simulink library "MagnetoLibrary"  (R2019a)
settings: Solver=VariableStepAuto  StartTime=0.0  StopTime=10.0  RelTol=1e-3
undefined symbols (not defined in the file or in its folder): quantity, Ts
libraries: arduinolib x8, $bdroot x4
settings Model: Creator=Jakub  LastModifiedBy=Jakub

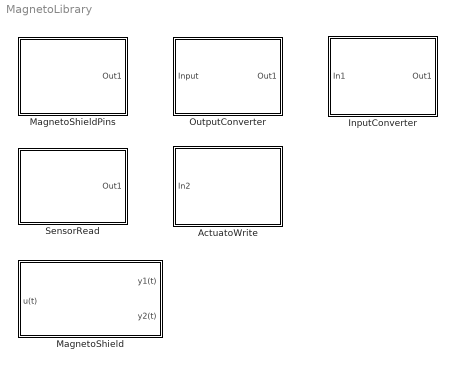
== system MagnetoLibrary ==
  ActuatoWrite : Subsystem  mask{Board=UNO/MEGA, Units=Volts}
      mask prompts: Board "Type of the Arduino board"; Units "Input unite"
      mask help:
      | ActuatorWrite block allows to set desired voltage value on the electromagnet. The desired value can be expresed as voltage, percentage of maximal possible voltage or as a value of the magnetic field in Gausses as well.
      | This block converts input control signal into suficient form (16-bit number) and writes the information on the MCP4725-DAC converter.
      | Maximal voltage range: 0-12 V
      mask init:
      | mask_popup = get_param(gcb,'Board'); % which popup is choosen
      | % path to the I2C Write block
      | system = gcb;
      | way = strcat(system,'/I2C Write UNO');
      | % set Module based on Arduino type
      | if strcmp(mask_popup(1),'U')
      |     set_param(way,'I2CModule','0'); % Uno/Mega - module 0
      | elseif strcmp(mask_popup(1),'D')
      |     set_param(way,'I2CModule','1'); % Due - module 1
      | end
      settings: CopyFcn=set_param(gcb, 'LinkStatus', 'inactive')
      mask TypeOptions Board: UNO/MEGA | DUE
      mask TypeOptions Units: Volts | Percents | DAC levels
      mask DialogControl DescGroupVar Prompt: ActuatorWrite block
      mask Display: image('assets\MagnetoFig\ActuatorWrite.bmp');
  InputConverter : Subsystem  mask{Units=Percents}
      mask prompts: Units "Choos input unit"
      mask help:
      | This block provide conversion between choosen input units and convert it into double number in range 0 to 4095. This converted size is suitable for "ActuatorWrite" block.
      | (input = double/output = double)
      mask init:
      | if Units==1
      | path = 'assets\MagnetoFig\InputCon\VtoDAC.bmp';
      | elseif Units==2
      | path = 'assets\MagnetoFig\InputCon\PERtoDAC.bmp';
      | else
      | path = 'assets\MagnetoFig\InputCon\DACtoDAC.bmp';    
      | end
      mask TypeOptions Units: Voltage | Percents | DAC levels
      mask DialogControl DescGroupVar Prompt: InputConverter block
      mask Display: image(path);
  MagnetoShield : Subsystem  mask{Board=UNO/MEGA, PositionType=Distance [mm], chackbox=on, Ts=0.001}
      mask prompts: Board "Type of the Arduino board"; PositionType "Position measured in:"; chackbox "Execute calibration at the biginning of the simulation"; Ts "Sampling period [s]"
      settings: CopyFcn=set_param(gcb, 'LinkStatus', 'inactive')
      mask TypeOptions Board: UNO/MEGA | DUE
      mask TypeOptions PositionType: Distance [mm] | Percents [%]
      mask DialogControl ParameterGroupVar Prompt: Arduino board
  MagnetoShieldPins : Subsystem  mask{PIN=Hall sensor pin (A3), sampling=0.001}
      mask prompts: PIN "Choose pin"; sampling "Sampling period [s]"
      mask help:
      | User can choose a pin on which the data should be processed.
      | >Hall sensor pin - data about the possition of the levitating magnet.
      | >Voltage pin - voltage on the electromagnet
      | >Current pin - current crossing the electromagnet
      | >Reference pin - data from potentiometer, used as adjustable analog reference
      | (output = double)
      mask init:
      | letter = PIN;
      | if letter==1
      | path='assets\MagnetoFig\Pins\hpin.bmp';
      | elseif letter==2
      | path='assets\MagnetoFig\Pins\vpin.bmp';
      | elseif letter==3
      | path='assets\MagnetoFig\Pins\cpin.bmp';
      | else
      | path='assets\MagnetoFig\Pins\ppin.bmp';    
      | end
      settings: CopyFcn=set_param(gcb, 'LinkStatus', 'inactive')
      mask TypeOptions PIN: Hall sensor pin (A3) | Voltage pin (A1) | Current pin (A2) | Reference pin (A0)
      mask Callback PIN:
      | mask_popup = get_param(gcb,'PIN'); % which popup is choosen
      | % path to the I2C Write block
      | system = gcb;
      | way = strcat(system,'/Analog Input');
      | % set Module based on Arduino type
      | if strcmp(mask_popup(1),'H')
      |     set_param(way,'pinNumber','3'); % Uno/Mega - module 0
      | elseif strcmp(mask_popup(1),'V')
      |     set_param(way,'pinNumber','1'); % Due - module 1
      | elseif strcmp(mask_popup(1),'C')
      |     set_param(way,'pinNumber','2'); % Due - module 1
      | elseif strcmp(mask_popup(1),'R')
      |     set_param(way,'pinNumber','0'); % Due - module 11
      | end
      mask DialogControl DescGroupVar Prompt: MagnetoShieldPins block
      mask Display: image(path);
  OutputConverter : Subsystem  mask{BoardType=UNO/MEGA, Units=Position, Pos=Distance, Dconst1=3.233100, Dconst2=0.220571, ADCmin_UNO=27, ADCmax_UNO=776, ADCmin_DUE=100, ADCmax_DUE=2315, ChackBox=off, VoltGain=4, CurrGain=33.333333, Parameter13=on}
      mask prompts: BoardType "Type of the Arduino board"; Units "Measured quantity"; Pos "Position unites"; Dconst1 "Position constant 1"; Dconst2 "Position constant 2"; ADCmin_UNO "Minimal ADC value uno"; ADCmax_UNO "Maximal  ADC value uno"; ADCmin_DUE "Minimal ADC value"; ADCmax_DUE "Maximal  ADC value"; ChackBox "Advanced options"; VoltGain "Voltage gain"; CurrGain "Current gain"; Parameter13 "Len pre funkcionalitu"
      mask help:
      | This block converts output signal from the system into choosen physical unit.
      | Entering signal is in the form of 8-bit number for Arduino UNO/MEGA or 12-bit number for Arduino DUE. Value on the output is defined by the choosen unit and possibly by the adjustnemts of these quantities.
      | Prefered input values from "MagnetoShieldPins" block.
      | (input = double/output = double)
      mask init:
      | if Units == 1 %position
      |         if Pos == 1 %mm
      |             path = 'assets\MagnetoFig\OutputCon\ADCtoMM.bmp'
      |         elseif Pos == 2 % percents
      |             path = 'assets\MagnetoFig\OutputCon\ADCtoPer.bmp'
      |         elseif Pos == 3 %gauss
      |            path = 'assets\MagnetoFig\OutputCon\ADCtoGauss.bmp' 
      |         else % adc levels
      |             path = 'assets\MagnetoFig\OutputCon\ADCtoADC.bmp'
      |         end
      |     elseif Units == 2 %voltage
      |         path = 'assets\MagnetoFig\OutputCon\ADCtoVolt.bmp'
      |     elseif Units == 3 %current
      |         path = 'assets\MagnetoFig\OutputCon\ADCtoAmp.bmp'
      |     else %analog reference
      |         path = 'assets\MagnetoFig\OutputCon\ADCtoRef.bmp'
      |     end
      mask TypeOptions BoardType: UNO/MEGA | DUE
      mask Callback BoardType:
      | mask_popup = get_param(gcb,'Units'); %Vyber meranej veliciny - Napatie/Prud/Poloha/Referencia
      | 
      | if strcmp(mask_popup(1),'P') %Ak meriam polohu
      |     set_param(gcb,'MaskVisibilities',{'on','on','on','off','off','off','off','off','off','off','off','off','off'});
      |     MeassurePos = get_param(gcb,'Pos'); %V com meriam polohu - Gauss/Vyska/Percenta/ADC
      |     if strcmp(MeassurePos(1),'D')
      |         set_param(gcb,'MaskVisibilities',{'on','on','on','on','on','off','off','off','off','off','off','off','off'});
      |     elseif strcmp(MeassurePos(1),'P')
      |         TypeOfBoard = get_param(gcb,'BoardType'); %Ak meriam v %, aku mam dosku?
      |         if strcmp(TypeOfBoard(1),'U')
      |             set_param(gcb,'MaskVisibilities',{'on','on','on','off','off','on','on','off','off','off','off','off','off'});
      |         else
      |             set_param(gcb,'MaskVisibilities',{'on','on','on','off','off','off','off','on','on','off','off','off','off'});
      |         end
      |     elseif strcmp(MeassurePos(1),'G')
      |         set_param(gcb,'MaskVisibilities',{'on','on','on','off','off','off','off','off','off','off','off','off','off'});
      |     else
      |         set_param(gcb,'MaskVisibilities',{'on','on','on','off','off','off','off','off','off','off','off','off','off'});
      |     end
      | elseif strcmp(mask_popup(1),'V') %Ak meriam napatie
      |     set_param(gcb,'MaskVisibilities',{'on','on','off','off','off','off','off','off','off','on','off','off','off'});
      |     mask_popupV = get_param(gcb,'ChackBox');
      |     if strcmp(mask_popupV(1),'o') & strcmp(mask_popupV(2),'n')%mask_popup == 'on'
      |         set_param(gcb,'MaskVisibilities',{'on','on','off','off','off','off','off','off','off','on','on','on','off'});
      |     else
      |         set_param(gcb,'MaskVisibilities',{'on','on','off','off','off','off','off','off','off','on','off','off','off'});
      |     end
      | elseif strcmp(mask_popup(1),'C') %Ak meriam prud
      |     set_param(gcb,'MaskVisibilities',{'on','on','off','off','off','off','off','off','off','on','off','off','off'});
      |     mask_popupC = get_param(gcb,'ChackBox');
      |     if strcmp(mask_popupC(1),'o') & strcmp(mask_popupC(2),'n')%mask_popup == 'on'
      |         set_param(gcb,'MaskVisibilities',{'on','on','off','off','off','off','off','off','off','on','on','on','off'});
      |     else
      |         set_param(gcb,'MaskVisibilities',{'on','on','off','off','off','off','off','off','off','on','off','off','off'});
      |     end
      | else %Ak meriam referenciu
      |     set_param(gcb,'MaskVisibilities',{'on','on','off','off','off','off','off','off','off','off','off','off','off'});
      | end
      mask TypeOptions Units: Position | Voltage [V] | Current [mA] | Analog reference [%]
      mask Callback Units:
      | mask_popup = get_param(gcb,'Units'); %Vyber meranej veliciny - Napatie/Prud/Poloha/Referencia
      | 
      | if strcmp(mask_popup(1),'P') %Ak meriam polohu
      |     set_param(gcb,'MaskVisibilities',{'on','on','on','off','off','off','off','off','off','off','off','off','off'});
      |     MeassurePos = get_param(gcb,'Pos'); %V com meriam polohu - Gauss/Vyska/Percenta/ADC
      |     if strcmp(MeassurePos(1),'D')
      |         set_param(gcb,'MaskVisibilities',{'on','on','on','on','on','off','off','off','off','off','off','off','off'});
      |     elseif strcmp(MeassurePos(1),'P')
      |         TypeOfBoard = get_param(gcb,'BoardType'); %Ak meriam v %, aku mam dosku?
      |         if strcmp(TypeOfBoard(1),'U')
      |             set_param(gcb,'MaskVisibilities',{'on','on','on','off','off','on','on','off','off','off','off','off','off'});
      |         else
      |             set_param(gcb,'MaskVisibilities',{'on','on','on','off','off','off','off','on','on','off','off','off','off'});
      |         end
      |     elseif strcmp(MeassurePos(1),'G')
      |         set_param(gcb,'MaskVisibilities',{'on','on','on','off','off','off','off','off','off','off','off','off','off'});
      |     else
      |         set_param(gcb,'MaskVisibilities',{'on','on','on','off','off','off','off','off','off','off','off','off','off'});
      |     end
      | elseif strcmp(mask_popup(1),'V') %Ak meriam napatie
      |     set_param(gcb,'MaskVisibilities',{'on','on','off','off','off','off','off','off','off','on','off','off','off'});
      |     mask_popupV = get_param(gcb,'ChackBox');
      |     if strcmp(mask_popupV(1),'o') & strcmp(mask_popupV(2),'n')%mask_popup == 'on'
      |         set_param(gcb,'MaskVisibilities',{'on','on','off','off','off','off','off','off','off','on','on','on','off'});
      |     else
      |         set_param(gcb,'MaskVisibilities',{'on','on','off','off','off','off','off','off','off','on','off','off','off'});
      |     end
      | elseif strcmp(mask_popup(1),'C') %Ak meriam prud
      |     set_param(gcb,'MaskVisibilities',{'on','on','off','off','off','off','off','off','off','on','off','off','off'});
      |     mask_popupC = get_param(gcb,'ChackBox');
      |     if strcmp(mask_popupC(1),'o') & strcmp(mask_popupC(2),'n')%mask_popup == 'on'
      |         set_param(gcb,'MaskVisibilities',{'on','on','off','off','off','off','off','off','off','on','on','on','off'});
      |     else
      |         set_param(gcb,'MaskVisibilities',{'on','on','off','off','off','off','off','off','off','on','off','off','off'});
      |     end
      | else %Ak meriam referenciu
      |     set_param(gcb,'MaskVisibilities',{'on','on','off','off','off','off','off','off','off','off','off','off','off'});
      | end
      mask TypeOptions Pos: Distance | Percents | Gauss | ADC levels
      mask Callback Pos:
      | MeassurePos = get_param(gcb,'Pos'); %V com meriam polohu - Gauss/Vyska/Percenta/ADC
      |     if strcmp(MeassurePos(1),'D')
      |         set_param(gcb,'MaskVisibilities',{'on','on','on','on','on','off','off','off','off','off','off','off','off'});
      |     elseif strcmp(MeassurePos(1),'P')
      |         TypeOfBoard = get_param(gcb,'BoardType'); %Ak meriam v %, aku mam dosku?
      |         if strcmp(TypeOfBoard(1),'U')
      |             set_param(gcb,'MaskVisibilities',{'on','on','on','off','off','on','on','off','off','off','off','off','off'});
      |         else
      |             set_param(gcb,'MaskVisibilities',{'on','on','on','off','off','off','off','on','on','off','off','off','off'});
      |         end
      |     elseif strcmp(MeassurePos(1),'G')
      |         set_param(gcb,'MaskVisibilities',{'on','on','on','off','off','off','off','off','off','off','off','off','off'});
      |     else
      |         set_param(gcb,'MaskVisibilities',{'on','on','on','off','off','off','off','off','off','off','off','off','off'});
      |     end
      mask Callback ChackBox:
      | mask_popup = get_param(gcb,'ChackBox');
      | 
      | if strcmp(mask_popup(1),'o') & strcmp(mask_popup(2),'n')%mask_popup == 'on'
      |     set_param(gcb,'MaskVisibilities',{'on','on','off','off','off','off','off','off','off','on','on','on','off'});
      | else
      |     set_param(gcb,'MaskVisibilities',{'on','on','off','off','off','off','off','off','off','on','off','off','off'});
      | end
      mask Callback Parameter13:
      | mask_popup = get_param(gcb,'Units'); %Vyber meranej veliciny - Napatie/Prud/Poloha/Referencia
      | 
      | if strcmp(mask_popup(1),'P') %Ak meriam polohu
      |     set_param(gcb,'MaskVisibilities',{'on','on','on','off','off','off','off','off','off','off','off','off','off'});
      |     MeassurePos = get_param(gcb,'Pos'); %V com meriam polohu - Gauss/Vyska/Percenta/ADC
      |     if strcmp(MeassurePos(1),'D')
      |         set_param(gcb,'MaskVisibilities',{'on','on','on','on','on','off','off','off','off','off','off','off','off'});
      |     elseif strcmp(MeassurePos(1),'P')
      |         TypeOfBoard = get_param(gcb,'BoardType'); %Ak meriam v %, aku mam dosku?
      |         if strcmp(TypeOfBoard(1),'U')
      |             set_param(gcb,'MaskVisibilities',{'on','on','on','off','off','on','on','off','off','off','off','off','off'});
      |         else
      |             set_param(gcb,'MaskVisibilities',{'on','on','on','off','off','off','off','on','on','off','off','off','off'});
      |         end
      |     elseif strcmp(MeassurePos(1),'G')
      |         set_param(gcb,'MaskVisibilities',{'on','on','on','off','off','off','off','off','off','off','off','off','off'});
      |     else
      |         set_param(gcb,'MaskVisibilities',{'on','on','on','off','off','off','off','off','off','off','off','off','off'});
      |     end
      | elseif strcmp(mask_popup(1),'V') %Ak meriam napatie
      |     set_param(gcb,'MaskVisibilities',{'on','on','off','off','off','off','off','off','off','on','off','off','off'});
      |     mask_popupV = get_param(gcb,'ChackBox');
      |     if strcmp(mask_popupV(1),'o') & strcmp(mask_popupV(2),'n')%mask_popup == 'on'
      |         set_param(gcb,'MaskVisibilities',{'on','on','off','off','off','off','off','off','off','on','on','on','off'});
      |     else
      |         set_param(gcb,'MaskVisibilities',{'on','on','off','off','off','off','off','off','off','on','off','off','off'});
      |     end
      | elseif strcmp(mask_popup(1),'C') %Ak meriam prud
      |     set_param(gcb,'MaskVisibilities',{'on','on','off','off','off','off','off','off','off','on','off','off','off'});
      |     mask_popupC = get_param(gcb,'ChackBox');
      |     if strcmp(mask_popupC(1),'o') & strcmp(mask_popupC(2),'n')%mask_popup == 'on'
      |         set_param(gcb,'MaskVisibilities',{'on','on','off','off','off','off','off','off','off','on','on','on','off'});
      |     else
      |         set_param(gcb,'MaskVisibilities',{'on','on','off','off','off','off','off','off','off','on','off','off','off'});
      |     end
      | else %Ak meriam referenciu
      |     set_param(gcb,'MaskVisibilities',{'on','on','off','off','off','off','off','off','off','off','off','off','off'});
      | end
      mask DialogControl DescGroupVar Prompt: OutputConverter block
      mask DialogControl ParameterGroupVar Prompt: Arduino board
      mask DialogControl Container3 Prompt: Parameters
      mask Display: image(path,'center');
  SensorRead : Subsystem  mask{board=UNO/MEGA, sensor=Distance [mm], sampling=0.001}
      mask prompts: board "Type of the Arduino board"; sensor "Sensor type"; sampling "Sampling period [s]"
      settings: CopyFcn=set_param(gcb, 'LinkStatus', 'inactive')
      mask TypeOptions board: UNO/MEGA | DUE
      mask TypeOptions sensor: Distance [mm] | Current [mA] | Voltage [V] | Analog reference [%]
      mask Callback sensor:
      | mask_popup = get_param(gcb,'sensor'); % which popup is choosen
      | % path to the I2C Write block
      | system = gcb;
      | way = strcat(system,'/Analog Input');
      | % set Module based on Arduino type
      | if strcmp(mask_popup(1),'D')
      |     set_param(way,'pinNumber','3');
      | elseif strcmp(mask_popup(1),'V')
      |     set_param(way,'pinNumber','1'); % Due - module 1
      | elseif strcmp(mask_popup(1),'C')
      |     set_param(way,'pinNumber','2'); % Due - module 1
      | elseif strcmp(mask_popup(1),'A')
      |     set_param(way,'pinNumber','0'); % Due - module 11
      | end
      mask DialogControl ParameterGroupVar Prompt: Arduino board

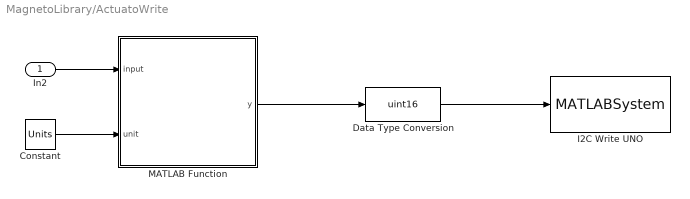
== system MagnetoLibrary/ActuatoWrite ==
  In2 : Inport
  Constant : Constant  Value=Units
  Data Type Conversion : DataTypeConversion  OutDataTypeStr=uint16
  I2C Write UNO : MATLABSystem  AncestorBlock=arduinolib/I2C Write  InitFcn=|  System=codertarget.arduinobase.internal.arduinoI2CWrite  I2CModule=0  Mode=Master  SlaveAddress=96  SlaveByteOrder=BigEndian  Direction=Transmitter  RegisterAddressMode=off  RegisterAddress=0  SlaveDataType=uint8  DataLength=1  NoAck=off  RepeatedStart=off  OutputStatus=off  blockPlatform=ARDUINO
      | codertarget.arduinobase.blocks.registerI2CBlock(gcbh);
      | codertarget.arduinobase.blocks.arduinoBlockInitFcnCallback(gcbh);
      mask Type: I2C Write
      mask Display:
      | color('white');
      | plot([100,100,100,100],[100,100,100,100]);
      | plot([0,0,0,0],[0,0,0,0]);
      | color('blue');
      | text(99, 92, 'ARDUINO', 'horizontalAlignment', 'right');
      | color('black');
      | text(50,60,'\fontsize{12}\bfI2C','texmode','on','horizontalAlignment','center','verticalAlignment','middle');
      | text(50,40,'\fontsize{10}\bfMaster Write','texmode','on','horizontalAlignment','center','verticalAlignment','middle');
      | text(50,15,'Slave: 0x60' ,'horizontalAlignment', 'center');
      | port_label('input',1,'Data');
  MATLAB Function : MATLAB Function  TreatAsAtomicUnit=on
  wires:
  In2/1 -> MATLAB Function/1(input)
  Constant/1 -> MATLAB Function/2(unit)
  Data Type Conversion/1 -> I2C Write UNO/1
  MATLAB Function/1(y) -> Data Type Conversion/1

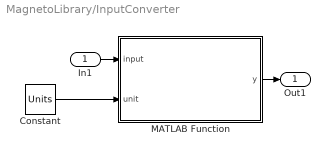
== system MagnetoLibrary/InputConverter ==
  In1 : Inport
  Constant : Constant  Value=Units
  MATLAB Function : MATLAB Function  TreatAsAtomicUnit=on
  Out1 : Outport
  wires:
  MATLAB Function/1(y) -> Out1/1
  Constant/1 -> MATLAB Function/2(unit)
  In1/1 -> MATLAB Function/1(input)

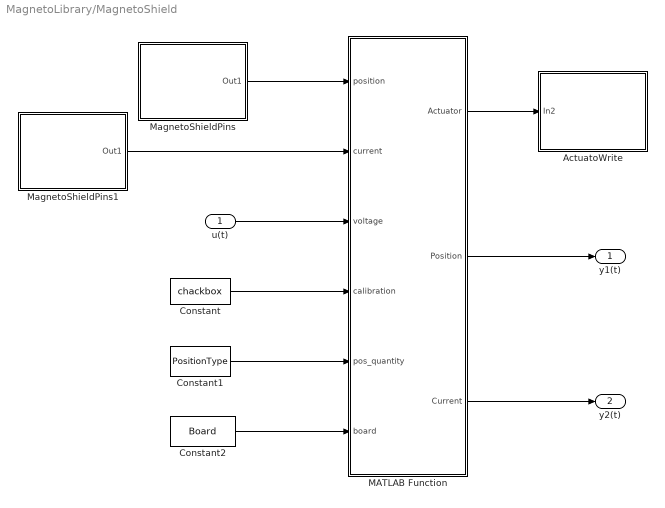
== system MagnetoLibrary/MagnetoShield ==
  u(t) : Inport
  ActuatoWrite : Subsystem  AncestorBlock=MagnetoLibrary/ActuatoWrite  mask{Board=DUE, Units=Volts}
      mask prompts: Board "Type of the Arduino board"; Units "Input unite"
      mask help:
      | ActuatorWrite block allows to set desired voltage value on the electromagnet. The desired value can be expresed as voltage, percentage of maximal possible voltage or as a value of the magnetic field in Gausses as well.
      | This block converts input control signal into suficient form (16-bit number) and writes the information on the MCP4725-DAC converter.
      | Maximal voltage range: 0-12 V
      mask init: same as MagnetoLibrary/ActuatoWrite
      settings: CopyFcn=set_param(gcb, 'LinkStatus', 'inactive')
      mask TypeOptions Board: UNO/MEGA | DUE
      mask TypeOptions Units: Volts | Percents | DAC levels
      mask DialogControl DescGroupVar Prompt: ActuatorWrite block
      mask Display: image('assets\MagnetoFig\ActuatorWrite.bmp');
  Constant : Constant  Value=chackbox  SampleTime=Ts
  Constant1 : Constant  Value=PositionType  SampleTime=Ts
  Constant2 : Constant  Value=Board  SampleTime=Ts
  MATLAB Function : MATLAB Function  TreatAsAtomicUnit=on
  MagnetoShieldPins : Subsystem  AncestorBlock=MagnetoLibrary/MagnetoShieldPins  mask{PIN=Hall sensor pin (A3), sampling=Ts}
      mask prompts: PIN "Choose pin"; sampling "Sampling period [s]"
      mask help:
      | User can choose a pin on which the data should be processed.
      | >Hall sensor pin - data about the possition of the levitating magnet.
      | >Voltage pin - voltage on the electromagnet
      | >Current pin - current crossing the electromagnet
      | >Reference pin - data from potentiometer, used as adjustable analog reference
      | (output = double)
      mask init: same as MagnetoLibrary/MagnetoShieldPins
      settings: CopyFcn=set_param(gcb, 'LinkStatus', 'inactive')
      mask TypeOptions PIN: Hall sensor pin (A3) | Voltage pin (A1) | Current pin (A2) | Reference pin (A0)
      mask Callback PIN:
      | mask_popup = get_param(gcb,'PIN'); % which popup is choosen
      | % path to the I2C Write block
      | system = gcb;
      | way = strcat(system,'/Analog Input');
      | % set Module based on Arduino type
      | if strcmp(mask_popup(1),'H')
      |     set_param(way,'pinNumber','3'); % Uno/Mega - module 0
      | elseif strcmp(mask_popup(1),'V')
      |     set_param(way,'pinNumber','1'); % Due - module 1
      | elseif strcmp(mask_popup(1),'C')
      |     set_param(way,'pinNumber','2'); % Due - module 1
      | elseif strcmp(mask_popup(1),'R')
      |     set_param(way,'pinNumber','0'); % Due - module 11
      | end
      mask DialogControl DescGroupVar Prompt: MagnetoShieldPins block
      mask Display: image(path);
  MagnetoShieldPins1 : Subsystem  AncestorBlock=MagnetoLibrary/MagnetoShieldPins  mask{PIN=Current pin (A2), sampling=Ts}
      mask prompts: PIN "Choose pin"; sampling "Sampling period [s]"
      mask help:
      | User can choose a pin on which the data should be processed.
      | >Hall sensor pin - data about the possition of the levitating magnet.
      | >Voltage pin - voltage on the electromagnet
      | >Current pin - current crossing the electromagnet
      | >Reference pin - data from potentiometer, used as adjustable analog reference
      | (output = double)
      mask init: same as MagnetoLibrary/MagnetoShieldPins
      settings: CopyFcn=set_param(gcb, 'LinkStatus', 'inactive')
      mask TypeOptions PIN: Hall sensor pin (A3) | Voltage pin (A1) | Current pin (A2) | Reference pin (A0)
      mask Callback PIN:
      | mask_popup = get_param(gcb,'PIN'); % which popup is choosen
      | % path to the I2C Write block
      | system = gcb;
      | way = strcat(system,'/Analog Input');
      | % set Module based on Arduino type
      | if strcmp(mask_popup(1),'H')
      |     set_param(way,'pinNumber','3'); % Uno/Mega - module 0
      | elseif strcmp(mask_popup(1),'V')
      |     set_param(way,'pinNumber','1'); % Due - module 1
      | elseif strcmp(mask_popup(1),'C')
      |     set_param(way,'pinNumber','2'); % Due - module 1
      | elseif strcmp(mask_popup(1),'R')
      |     set_param(way,'pinNumber','0'); % Due - module 11
      | end
      mask DialogControl DescGroupVar Prompt: MagnetoShieldPins block
      mask Display: image(path);
  y1(t) : Outport
  y2(t) : Outport  Port=2
  wires:
  MATLAB Function/3(Current) -> y2(t)/1
  Constant2/1 -> MATLAB Function/6(board)
  Constant1/1 -> MATLAB Function/5(pos_quantity)
  Constant/1 -> MATLAB Function/4(calibration)
  MagnetoShieldPins1/1(Out1) -> MATLAB Function/2(current)
  u(t)/1 -> MATLAB Function/3(voltage)
  MATLAB Function/2(Position) -> y1(t)/1
  MagnetoShieldPins/1(Out1) -> MATLAB Function/1(position)
  MATLAB Function/1(Actuator) -> ActuatoWrite/1(In2)

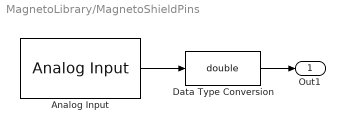
== system MagnetoLibrary/MagnetoShieldPins ==
  Analog Input : arduinolib/Analog Input  pinNumber=3  ReadResultsOnly=off  ConversionTriggerSource=Software  ExternalTriggerType=uint32(0)  OutputDataType=uint16  EnableConversionCompleteNotify=off  EnableOuputStatus=off  SampleTime=sampling  blockPlatform=arduino
  Data Type Conversion : DataTypeConversion  OutDataTypeStr=double
  Out1 : Outport
  wires:
  Analog Input/1 -> Data Type Conversion/1
  Data Type Conversion/1 -> Out1/1

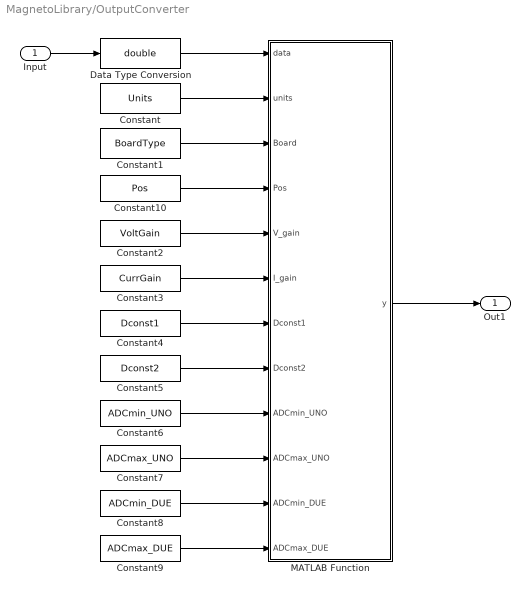
== system MagnetoLibrary/OutputConverter ==
  Input : Inport
  Constant : Constant  Value=Units
  Constant1 : Constant  Value=BoardType
  Constant10 : Constant  Value=Pos
  Constant2 : Constant  Value=VoltGain
  Constant3 : Constant  Value=CurrGain
  Constant4 : Constant  Value=Dconst1
  Constant5 : Constant  Value=Dconst2
  Constant6 : Constant  Value=ADCmin_UNO
  Constant7 : Constant  Value=ADCmax_UNO
  Constant8 : Constant  Value=ADCmin_DUE
  Constant9 : Constant  Value=ADCmax_DUE
  Data Type Conversion : DataTypeConversion  OutDataTypeStr=double
  MATLAB Function : MATLAB Function  TreatAsAtomicUnit=on
  Out1 : Outport
  wires:
  Constant4/1 -> MATLAB Function/7(Dconst1)
  Constant5/1 -> MATLAB Function/8(Dconst2)
  Constant6/1 -> MATLAB Function/9(ADCmin_UNO)
  Constant7/1 -> MATLAB Function/10(ADCmax_UNO)
  Constant8/1 -> MATLAB Function/11(ADCmin_DUE)
  Constant9/1 -> MATLAB Function/12(ADCmax_DUE)
  Data Type Conversion/1 -> MATLAB Function/1(data)
  Constant3/1 -> MATLAB Function/6(I_gain)
  Constant2/1 -> MATLAB Function/5(V_gain)
  Constant1/1 -> MATLAB Function/3(Board)
  Constant/1 -> MATLAB Function/2(units)
  MATLAB Function/1(y) -> Out1/1
  Input/1 -> Data Type Conversion/1
  Constant10/1 -> MATLAB Function/4(Pos)

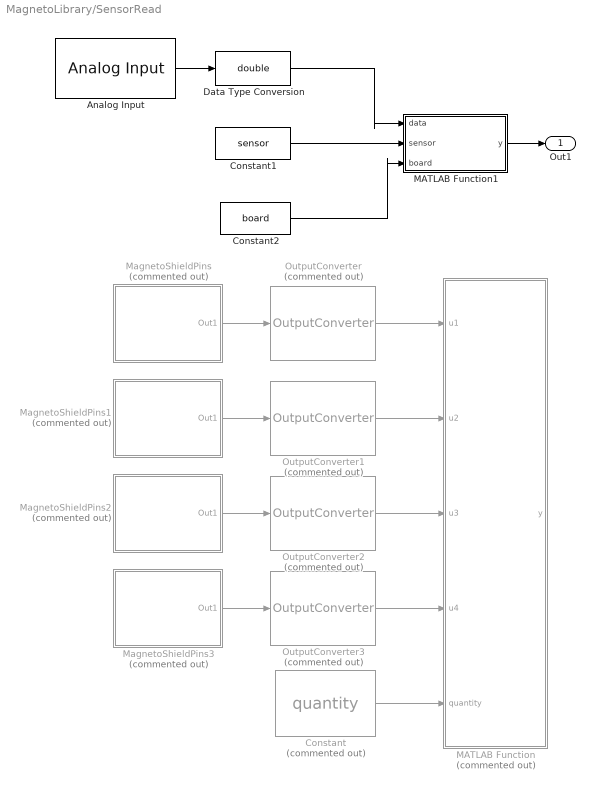
== system MagnetoLibrary/SensorRead ==
  Analog Input : arduinolib/Analog Input  pinNumber=3  ReadResultsOnly=off  ConversionTriggerSource=Software  ExternalTriggerType=uint32(0)  OutputDataType=uint16  EnableConversionCompleteNotify=off  EnableOuputStatus=off  SampleTime=sampling  blockPlatform=arduino
  Constant : Constant  Commented=on  Value=quantity  SampleTime=Ts
  Constant1 : Constant  Value=sensor
  Constant2 : Constant  Value=board
  Data Type Conversion : DataTypeConversion  OutDataTypeStr=double
  MATLAB Function : MATLAB Function  Commented=on  TreatAsAtomicUnit=on
  MATLAB Function1 : MATLAB Function  TreatAsAtomicUnit=on
  MagnetoShieldPins : Subsystem  Commented=on  AncestorBlock=MagnetoLibrary/MagnetoShieldPins  mask{PIN=Hall sensor pin (A3), sampling=Ts}
      mask prompts: PIN "Choose pin"; sampling "Sampling period [s]"
      mask help:
      | User can choose a pin on which the data should be processed.
      | >Hall sensor pin - data about the possition of the levitating magnet.
      | >Voltage pin - voltage on the electromagnet
      | >Current pin - current crossing the electromagnet
      | >Reference pin - data from potentiometer, used as adjustable analog reference
      | (output = double)
      mask init: same as MagnetoLibrary/MagnetoShieldPins
      settings: CopyFcn=set_param(gcb, 'LinkStatus', 'inactive')
      mask TypeOptions PIN: Hall sensor pin (A3) | Voltage pin (A1) | Current pin (A2) | Reference pin (A0)
      mask Callback PIN:
      | mask_popup = get_param(gcb,'PIN'); % which popup is choosen
      | % path to the I2C Write block
      | system = gcb;
      | way = strcat(system,'/Analog Input');
      | % set Module based on Arduino type
      | if strcmp(mask_popup(1),'H')
      |     set_param(way,'pinNumber','3'); % Uno/Mega - module 0
      | elseif strcmp(mask_popup(1),'V')
      |     set_param(way,'pinNumber','1'); % Due - module 1
      | elseif strcmp(mask_popup(1),'C')
      |     set_param(way,'pinNumber','2'); % Due - module 1
      | elseif strcmp(mask_popup(1),'R')
      |     set_param(way,'pinNumber','0'); % Due - module 11
      | end
      mask DialogControl DescGroupVar Prompt: MagnetoShieldPins block
      mask Display: image(path);
  MagnetoShieldPins1 : Subsystem  Commented=on  AncestorBlock=MagnetoLibrary/MagnetoShieldPins  mask{PIN=Current pin (A2), sampling=Ts}
      mask prompts: PIN "Choose pin"; sampling "Sampling period [s]"
      mask help:
      | User can choose a pin on which the data should be processed.
      | >Hall sensor pin - data about the possition of the levitating magnet.
      | >Voltage pin - voltage on the electromagnet
      | >Current pin - current crossing the electromagnet
      | >Reference pin - data from potentiometer, used as adjustable analog reference
      | (output = double)
      mask init: same as MagnetoLibrary/MagnetoShieldPins
      settings: CopyFcn=set_param(gcb, 'LinkStatus', 'inactive')
      mask TypeOptions PIN: Hall sensor pin (A3) | Voltage pin (A1) | Current pin (A2) | Reference pin (A0)
      mask Callback PIN:
      | mask_popup = get_param(gcb,'PIN'); % which popup is choosen
      | % path to the I2C Write block
      | system = gcb;
      | way = strcat(system,'/Analog Input');
      | % set Module based on Arduino type
      | if strcmp(mask_popup(1),'H')
      |     set_param(way,'pinNumber','3'); % Uno/Mega - module 0
      | elseif strcmp(mask_popup(1),'V')
      |     set_param(way,'pinNumber','1'); % Due - module 1
      | elseif strcmp(mask_popup(1),'C')
      |     set_param(way,'pinNumber','2'); % Due - module 1
      | elseif strcmp(mask_popup(1),'R')
      |     set_param(way,'pinNumber','0'); % Due - module 11
      | end
      mask DialogControl DescGroupVar Prompt: MagnetoShieldPins block
      mask Display: image(path);
  MagnetoShieldPins2 : Subsystem  Commented=on  AncestorBlock=MagnetoLibrary/MagnetoShieldPins  mask{PIN=Voltage pin (A1), sampling=Ts}
      mask prompts: PIN "Choose pin"; sampling "Sampling period [s]"
      mask help:
      | User can choose a pin on which the data should be processed.
      | >Hall sensor pin - data about the possition of the levitating magnet.
      | >Voltage pin - voltage on the electromagnet
      | >Current pin - current crossing the electromagnet
      | >Reference pin - data from potentiometer, used as adjustable analog reference
      | (output = double)
      mask init: same as MagnetoLibrary/MagnetoShieldPins
      settings: CopyFcn=set_param(gcb, 'LinkStatus', 'inactive')
      mask TypeOptions PIN: Hall sensor pin (A3) | Voltage pin (A1) | Current pin (A2) | Reference pin (A0)
      mask Callback PIN:
      | mask_popup = get_param(gcb,'PIN'); % which popup is choosen
      | % path to the I2C Write block
      | system = gcb;
      | way = strcat(system,'/Analog Input');
      | % set Module based on Arduino type
      | if strcmp(mask_popup(1),'H')
      |     set_param(way,'pinNumber','3'); % Uno/Mega - module 0
      | elseif strcmp(mask_popup(1),'V')
      |     set_param(way,'pinNumber','1'); % Due - module 1
      | elseif strcmp(mask_popup(1),'C')
      |     set_param(way,'pinNumber','2'); % Due - module 1
      | elseif strcmp(mask_popup(1),'R')
      |     set_param(way,'pinNumber','0'); % Due - module 11
      | end
      mask DialogControl DescGroupVar Prompt: MagnetoShieldPins block
      mask Display: image(path);
  MagnetoShieldPins3 : Subsystem  Commented=on  AncestorBlock=MagnetoLibrary/MagnetoShieldPins  mask{PIN=Reference pin (A0), sampling=Ts}
      mask prompts: PIN "Choose pin"; sampling "Sampling period [s]"
      mask help:
      | User can choose a pin on which the data should be processed.
      | >Hall sensor pin - data about the possition of the levitating magnet.
      | >Voltage pin - voltage on the electromagnet
      | >Current pin - current crossing the electromagnet
      | >Reference pin - data from potentiometer, used as adjustable analog reference
      | (output = double)
      mask init: same as MagnetoLibrary/MagnetoShieldPins
      settings: CopyFcn=set_param(gcb, 'LinkStatus', 'inactive')
      mask TypeOptions PIN: Hall sensor pin (A3) | Voltage pin (A1) | Current pin (A2) | Reference pin (A0)
      mask Callback PIN:
      | mask_popup = get_param(gcb,'PIN'); % which popup is choosen
      | % path to the I2C Write block
      | system = gcb;
      | way = strcat(system,'/Analog Input');
      | % set Module based on Arduino type
      | if strcmp(mask_popup(1),'H')
      |     set_param(way,'pinNumber','3'); % Uno/Mega - module 0
      | elseif strcmp(mask_popup(1),'V')
      |     set_param(way,'pinNumber','1'); % Due - module 1
      | elseif strcmp(mask_popup(1),'C')
      |     set_param(way,'pinNumber','2'); % Due - module 1
      | elseif strcmp(mask_popup(1),'R')
      |     set_param(way,'pinNumber','0'); % Due - module 11
      | end
      mask DialogControl DescGroupVar Prompt: MagnetoShieldPins block
      mask Display: image(path);
  OutputConverter : $bdroot/OutputConverter  Commented=on  BoardType=DUE  Units=Position  Pos=Distance  Dconst1=3.233100  Dconst2=0.220571  ADCmin_UNO=27  ADCmax_UNO=776  ADCmin_DUE=100  ADCmax_DUE=2315  ChackBox=off  VoltGain=4  CurrGain=33.333333  Parameter13=on
  OutputConverter1 : $bdroot/OutputConverter  Commented=on  BoardType=DUE  Units=Current [mA]  Pos=Distance  Dconst1=3.233100  Dconst2=0.220571  ADCmin_UNO=27  ADCmax_UNO=776  ADCmin_DUE=100  ADCmax_DUE=2315  ChackBox=off  VoltGain=4  CurrGain=33.333333  Parameter13=on
  OutputConverter2 : $bdroot/OutputConverter  Commented=on  BoardType=DUE  Units=Voltage [V]  Pos=Distance  Dconst1=3.233100  Dconst2=0.220571  ADCmin_UNO=27  ADCmax_UNO=776  ADCmin_DUE=100  ADCmax_DUE=2315  ChackBox=off  VoltGain=4  CurrGain=33.333333  Parameter13=on
  OutputConverter3 : $bdroot/OutputConverter  Commented=on  BoardType=DUE  Units=Analog reference [%]  Pos=Distance  Dconst1=3.233100  Dconst2=0.220571  ADCmin_UNO=27  ADCmax_UNO=776  ADCmin_DUE=100  ADCmax_DUE=2315  ChackBox=off  VoltGain=4  CurrGain=33.333333  Parameter13=on
  Out1 : Outport
  wires:
  Constant2/1 -> MATLAB Function1/3(board)
  Constant1/1 -> MATLAB Function1/2(sensor)
  MATLAB Function1/1(y) -> Out1/1
  MagnetoShieldPins1/1(Out1) -> OutputConverter1/1
  OutputConverter3/1 -> MATLAB Function/4(u4)
  MagnetoShieldPins3/1(Out1) -> OutputConverter3/1
  OutputConverter/1 -> MATLAB Function/1(u1)
  MagnetoShieldPins2/1(Out1) -> OutputConverter2/1
  MagnetoShieldPins/1(Out1) -> OutputConverter/1
  OutputConverter1/1 -> MATLAB Function/2(u2)
  OutputConverter2/1 -> MATLAB Function/3(u3)
  Constant/1 -> MATLAB Function/5(quantity)
  Data Type Conversion/1 -> MATLAB Function1/1(data)
  Analog Input/1 -> Data Type Conversion/1

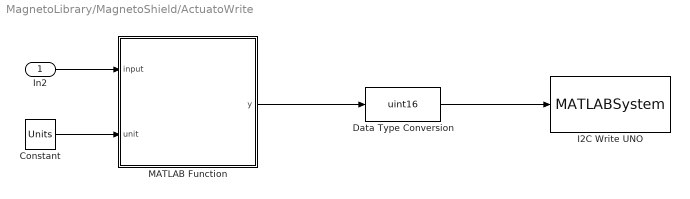
== system MagnetoLibrary/MagnetoShield/ActuatoWrite ==
  In2 : Inport
  Constant : Constant  Value=Units
  Data Type Conversion : DataTypeConversion  OutDataTypeStr=uint16
  I2C Write UNO : MATLABSystem  AncestorBlock=arduinolib/I2C Write  InitFcn=|  System=codertarget.arduinobase.internal.arduinoI2CWrite  I2CModule=1  Mode=Master  SlaveAddress=96  SlaveByteOrder=BigEndian  Direction=Transmitter  RegisterAddressMode=off  RegisterAddress=0  SlaveDataType=uint8  DataLength=1  NoAck=off  RepeatedStart=off  OutputStatus=off  blockPlatform=ARDUINO
      | codertarget.arduinobase.blocks.registerI2CBlock(gcbh);
      | codertarget.arduinobase.blocks.arduinoBlockInitFcnCallback(gcbh);
      mask Type: I2C Write
      mask Display:
      | color('white');
      | plot([100,100,100,100],[100,100,100,100]);
      | plot([0,0,0,0],[0,0,0,0]);
      | color('blue');
      | text(99, 92, 'ARDUINO', 'horizontalAlignment', 'right');
      | color('black');
      | text(50,60,'\fontsize{12}\bfI2C','texmode','on','horizontalAlignment','center','verticalAlignment','middle');
      | text(50,40,'\fontsize{10}\bfMaster Write','texmode','on','horizontalAlignment','center','verticalAlignment','middle');
      | text(50,15,'Slave: 0x60' ,'horizontalAlignment', 'center');
      | port_label('input',1,'Data');
  MATLAB Function : MATLAB Function  TreatAsAtomicUnit=on
  wires:
  In2/1 -> MATLAB Function/1(input)
  Constant/1 -> MATLAB Function/2(unit)
  Data Type Conversion/1 -> I2C Write UNO/1
  MATLAB Function/1(y) -> Data Type Conversion/1

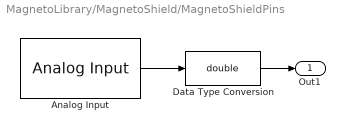
== system MagnetoLibrary/MagnetoShield/MagnetoShieldPins ==
  Analog Input : arduinolib/Analog Input  pinNumber=3  ReadResultsOnly=off  ConversionTriggerSource=Software  ExternalTriggerType=uint32(0)  OutputDataType=uint16  EnableConversionCompleteNotify=off  EnableOuputStatus=off  SampleTime=sampling  blockPlatform=arduino
  Data Type Conversion : DataTypeConversion  OutDataTypeStr=double
  Out1 : Outport
  wires:
  Analog Input/1 -> Data Type Conversion/1
  Data Type Conversion/1 -> Out1/1

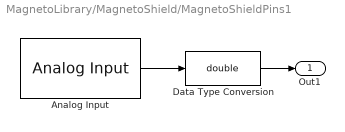
== system MagnetoLibrary/MagnetoShield/MagnetoShieldPins1 ==
  Analog Input : arduinolib/Analog Input  pinNumber=2  ReadResultsOnly=off  ConversionTriggerSource=Software  ExternalTriggerType=uint32(0)  OutputDataType=uint16  EnableConversionCompleteNotify=off  EnableOuputStatus=off  SampleTime=sampling  blockPlatform=arduino
  Data Type Conversion : DataTypeConversion  OutDataTypeStr=double
  Out1 : Outport
  wires:
  Analog Input/1 -> Data Type Conversion/1
  Data Type Conversion/1 -> Out1/1

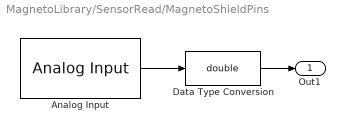
== system MagnetoLibrary/SensorRead/MagnetoShieldPins ==
  Analog Input : arduinolib/Analog Input  pinNumber=3  ReadResultsOnly=off  ConversionTriggerSource=Software  ExternalTriggerType=uint32(0)  OutputDataType=uint16  EnableConversionCompleteNotify=off  EnableOuputStatus=off  SampleTime=sampling  blockPlatform=arduino
  Data Type Conversion : DataTypeConversion  OutDataTypeStr=double
  Out1 : Outport
  wires:
  Analog Input/1 -> Data Type Conversion/1
  Data Type Conversion/1 -> Out1/1

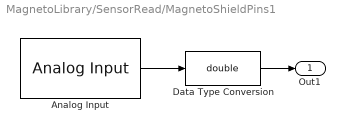
== system MagnetoLibrary/SensorRead/MagnetoShieldPins1 ==
  Analog Input : arduinolib/Analog Input  pinNumber=2  ReadResultsOnly=off  ConversionTriggerSource=Software  ExternalTriggerType=uint32(0)  OutputDataType=uint16  EnableConversionCompleteNotify=off  EnableOuputStatus=off  SampleTime=sampling  blockPlatform=arduino
  Data Type Conversion : DataTypeConversion  OutDataTypeStr=double
  Out1 : Outport
  wires:
  Analog Input/1 -> Data Type Conversion/1
  Data Type Conversion/1 -> Out1/1

== system MagnetoLibrary/SensorRead/MagnetoShieldPins2 ==
  Analog Input : arduinolib/Analog Input  pinNumber=1  ReadResultsOnly=off  ConversionTriggerSource=Software  ExternalTriggerType=uint32(0)  OutputDataType=uint16  EnableConversionCompleteNotify=off  EnableOuputStatus=off  SampleTime=sampling  blockPlatform=arduino
  Data Type Conversion : DataTypeConversion  OutDataTypeStr=double
  Out1 : Outport
  wires:
  Analog Input/1 -> Data Type Conversion/1
  Data Type Conversion/1 -> Out1/1

== system MagnetoLibrary/SensorRead/MagnetoShieldPins3 ==
  Analog Input : arduinolib/Analog Input  pinNumber=0  ReadResultsOnly=off  ConversionTriggerSource=Software  ExternalTriggerType=uint32(0)  OutputDataType=uint16  EnableConversionCompleteNotify=off  EnableOuputStatus=off  SampleTime=sampling  blockPlatform=arduino
  Data Type Conversion : DataTypeConversion  OutDataTypeStr=double
  Out1 : Outport
  wires:
  Analog Input/1 -> Data Type Conversion/1
  Data Type Conversion/1 -> Out1/1

== matlab function MagnetoLibrary/InputConverter/MATLAB Function ==
  data: input input; y output; unit input
function y = fcn(input,unit)

if unit==1 % voltage
    y = 4095/5*input;
elseif unit==2 % percents
    y = 4095/100*input;
elseif unit==3 % dac levels
    y = input;
else
     y = 0; % needed instance
end
% secures that 12-bit number will not overcross a size boundary
if y>4095
    y=4095;
elseif y<0
    y=0;
end

end

== matlab function MagnetoLibrary/SensorRead/MATLAB Function ==
  data: u1 input; y output; u2 input; u3 input; u4 input; quantity input
function y = fcn(u1,u2,u3,u4,quantity)
if quantity == 1
    y = u1;
elseif quantity == 2
    y = u2;
elseif quantity == 3
    y = u3; 
else %quantity == 4
    y = u4;
end

== matlab function MagnetoLibrary/ActuatoWrite/MATLAB Function ==
  data: input input; y output; unit input
function y = fcn(input,unit)

if unit==1 % voltage
    y = 4095/12*input;
elseif unit==2 % percents
    y = 4095/100*input;
elseif unit==3 % dac levels
    y = input;
else
     y = 0; % needed instance
end
% secures that 12-bit number will not overcross a size boundary
if y>4095
    y=4095;
elseif y<0
    y=0;
end

end

== matlab function MagnetoLibrary/OutputConverter/MATLAB Function ==
  data: data input; y output; units input; Board input; Pos input; V_gain input; I_gain input; Dconst1 input; Dconst2 input; ADCmin_UNO input; ADCmax_UNO input; ADCmin_DUE input; ADCmax_DUE input
function y = fcn(data,units,Board,Pos,V_gain,I_gain,Dconst1,Dconst2,ADCmin_UNO,...
    ADCmax_UNO,ADCmin_DUE,ADCmax_DUE)
A1302_SENSITIVITY = 769.23;
if Board==1
    ARES3V3 = 3.3/1023; % ADC constant for AVR architecture
elseif Board==2
    ARES3V3 = 3.3/4095; % ADC constant for SAM/SAMD architecture
else
    ARES3V3 = 0; % hase to be as a default case for successful compilation
end

if units==4 % Analog (Potentiometer) reference
    y = data*ARES3V3*100/3.3; % converts to '%'
elseif units==2 % Voltage
    y = data*ARES3V3*V_gain;
elseif units==3 % Current
    y = data*ARES3V3*I_gain;
elseif units==1 % Position
    if Pos == 1 % Distance
        gauss = (2.5-data*ARES3V3)*A1302_SENSITIVITY;
        y = Dconst1*gauss^Dconst2; % gauss to distance relationship
    elseif Pos == 2 % Percents
        if Board == 1
            maxV = ADCmax_UNO;
            minV = ADCmin_UNO;
        else
            maxV = ADCmax_DUE;
            minV = ADCmin_DUE;
        end
         y = (data-minV)*100/(maxV-minV);
    elseif Pos == 3 % Gausses
        y = (2.5-data*ARES3V3)*A1302_SENSITIVITY;
    else % ADC levels
        y = data;
    end
else
    y=0;
end

== matlab function MagnetoLibrary/SensorRead/MATLAB Function1 ==
  data: data input; y output; sensor input; board input
function y = fcn(data,sensor,board)
persistent init A1302_SENSITIVITY Dconst1 Dconst2 I_gain V_gain ARES3V3;
if isempty(init)
    init = 1;
    A1302_SENSITIVITY = 769.23;
    Dconst1 = 3.233100;
    Dconst2 = 0.220571;
    I_gain = 33.333333;
    V_gain = 4;
    if board==1
        ARES3V3 = 3.3/1023; % ADC constant for AVR architecture
    else
        ARES3V3 = 3.3/4095; % ADC constant for SAM/SAMD architecture
    end
end

if sensor==1                    % position
    gauss = (2.5-data*ARES3V3)*A1302_SENSITIVITY;
    y = Dconst1*gauss^Dconst2;
elseif sensor==2                % current
    y = data*ARES3V3*I_gain;
elseif sensor==3                % voltage
    y = data*ARES3V3*V_gain;
else                            % analog reference
    y = data*ARES3V3*100/3.3;
end

== matlab function MagnetoLibrary/MagnetoShield/ActuatoWrite/MATLAB Function ==
  data: input input; y output; unit input
function y = fcn(input,unit)

if unit==1 % voltage
    y = 4095/12*input;
elseif unit==2 % percents
    y = 4095/100*input;
elseif unit==3 % dac levels
    y = input;
else
     y = 0; % needed instance
end
% secures that 12-bit number will not overcross a size boundary
if y>4095
    y=4095;
elseif y<0
    y=0;
end

end

== matlab function MagnetoLibrary/MagnetoShield/MATLAB Function ==
  data: position input; Actuator output; current input; Position output; voltage input; calibration input; Current output; pos_quantity input; board input
function [Actuator,Position,Current] = fcn(position,current,voltage,calibration,pos_quantity,board)
persistent adcMAX adcMIN p_d1 p_d2 counter calib;
if isempty(counter)
         p_d1 = 3.233100;
         p_d2 = 0.220571;
         counter = 0;
         adcMAX = 300;
         adcMIN = 300;
         calib = calibration;
end
% CALIBRATION PHASE
if calib == 1
    % Minimal ADC level measured on the hall sensor
    if counter<=500
        Actuator = 0;
        if position<adcMIN
            adcMIN = position;
        end
    % Maximal ADC level measured on the hall sensor    
    elseif counter>500 && counter<=1000
        Actuator = 12;
        if position>adcMAX
            adcMAX = position; 
        end
    % Calibration calculations
    else
        Actuator = 0;
        p_d2 = log(17/12)/log((2.5-adcMIN*3.3/4095)*769.23/((2.5-adcMAX*3.3/4095)*769.23));
        p_d1 = 12/((2.5-adcMAX*3.3/4095)*769.23)^p_d2;
        % Time 500 samples to settle down the magnet
        if counter>1500
            calib = 0;
        end
    end
    Position = 0;   % default outputs during calibration
    Current = 0;
    counter = counter+1;
% CONTROL PHASE
elseif calib == 0
    Actuator = voltage;
    if board==1                 % choose board
        ARES3V3 = 3.3/1023;     % UNO
    elseif board==2
        ARES3V3 = 3.3/4095;     % DUE
    else
        ARES3V3 = 0;
    end
    % position measured in:
    if pos_quantity==2  % percents
        Position = (position-adcMIN)*100/(adcMAX-adcMIN);
    else            % distance
        gauss = (2.5-position*ARES3V3)*769.23; %A1302_SENSITIVITY = 769.23;
        Position = p_d1*gauss^p_d2;
    end
    % current measurement
    Current = current*ARES3V3*33.333333; %Igain = 33.333333
% ERROR SIGNALIZATION    
else
    Actuator = 42;
    Position = 42;
    Current = 42;
end
